simulink model "actrec_export"  (R2013a)
settings: Solver=FixedStepDiscrete  SolverMode=SingleTasking  StartTime=0  StopTime=220  RelTol=1e-3
libraries: simulink x2, dspsigops x2, dspstat3 x2, dspspect3 x2
settings Model: Creator=laurenz  LastModifiedBy=laurenz
settings OptimizationCC: OptimizeModelRefInitCode=on  LifeSpan=1
settings HardwareCC: ProdLargestAtomicInteger=Long  ProdLargestAtomicFloat=Double  ProdEndianess=LittleEndian  ProdHWDeviceType=ARM Compatible->ARM Cortex  TargetLargestAtomicInteger=Long  TargetLargestAtomicFloat=Double  TargetEndianess=LittleEndian  TargetHWDeviceType=ARM Compatible->ARM Cortex
settings RTWCC: SystemTargetFile=ert.tlc  GenCodeOnly=on  GenerateMakefile=off  TemplateMakefile=ert_default_tmf  Description=Embedded Coder  ProcessScript=ert_make_rtw_hook
settings CodeAppCC: IgnoreCustomStorageClasses=off
settings ERTTargetCC: GenerateSampleERTMain=off  IncludeMdlTerminateFcn=off  IncludeFileDelimiter=UseQuote  InlinedParameterPlacement=Hierarchical  ERTCustomFileTemplate=example_file_process.tlc  GlobalDataDefinition=InSourceFile  GlobalDataReference=InSourceFile  ERTFilePackagingFormat=Compact

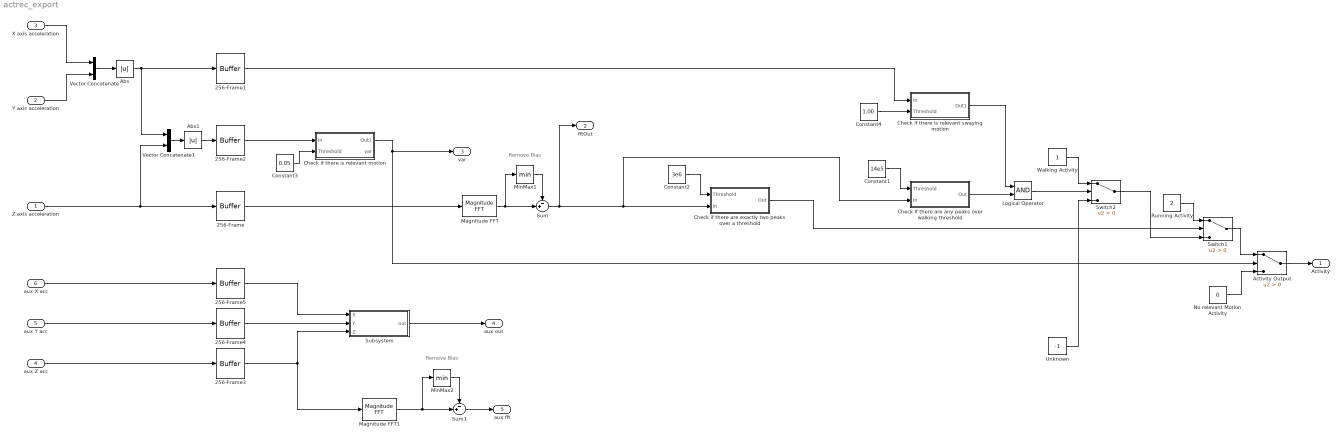
== system actrec_export ==
  note: Remove Bias
  note: Remove Bias
  Z axis acceleration : Inport  SampleTime=1
  Y axis acceleration : Inport  Port=2  SampleTime=1
  X axis acceleration : Inport  Port=3  SampleTime=1
  aux Z acc : Inport  Port=4  SampleTime=1
  aux Y acc : Inport  Port=5  SampleTime=1
  aux X acc : Inport  Port=6  SampleTime=1
  256-Frame{,1..5} (6 alike) : Buffer  N=256  V=256-64  TreatMby1Signals=One channel
  Abs : Abs
  Abs1 : Abs
  Activity Output : Switch  Criteria=u2 > Threshold
  Check if there are any peaks over walking threshold : Subsystem
  Check if there are exactly two peaks over a threshold : Subsystem
  Check if there is relevant motion : Subsystem
  Check if there is relevant swaying motion : Subsystem
  Constant1 : Constant  Value=14e5
  Constant2 : Constant  Value=3e6
  Constant3 : Constant  Value=0.05
  Constant4 : Constant  Value=1.00
  Logical Operator : Logic  AllPortsSameDT=off  OutDataTypeStr=boolean
  Magnitude FFT : dspspect3/Magnitude FFT  mag_or_magsq=Magnitude squared  FFTImplementation=Auto  fftLenInherit=on  fftsize=256
  Magnitude FFT1 : dspspect3/Magnitude FFT  mag_or_magsq=Magnitude squared  FFTImplementation=Auto  fftLenInherit=on  fftsize=256
  MinMax1 : MinMax
  MinMax2 : MinMax
  No relevant Motion Activity : Constant  Value=0
  Running Activity : Constant  Value=2
  Subsystem : Subsystem
  Sum : Sum  Inputs=-+|
  Sum1 : Sum  Inputs=-+|
  Switch1 : Switch  Criteria=u2 > Threshold
  Switch2 : Switch  Criteria=u2 > Threshold
  Unknown : Constant  Value=-1
  Vector Concatenate : Concatenate
  Vector Concatenate1 : Concatenate
  Walking Activity : Constant
  Activity : Outport
  fftOut : Outport  Port=2  PortDimensions=256
  var : Outport  Port=3
  aux out : Outport  Port=4
  aux fft : Outport  Port=5
  wires:
  Z axis acceleration/1 -> Vector Concatenate1/2, 256-Frame/1
  Activity Output/1 -> Activity/1
  No relevant Motion Activity/1 -> Activity Output/3
  Magnitude FFT/1 -> Sum/2, MinMax1/1
  MinMax1/1 -> Sum/1
  Check if there are exactly two peaks over a threshold/1(Out) -> Switch1/2
  Constant2/1 -> Check if there are exactly two peaks over a threshold/1(Threshold)
  Running Activity/1 -> Switch1/1
  Switch1/1 -> Activity Output/1
  Constant1/1 -> Check if there are any peaks over walking threshold/1(Threshold)
  Switch2/1 -> Switch1/3
  Walking Activity/1 -> Switch2/1
  Logical Operator/1 -> Switch2/2
  Check if there are any peaks over walking threshold/1(Out) -> Logical Operator/2
  Check if there is relevant swaying motion/1(Out1) -> Logical Operator/1
  Abs/1 -> 256-Frame1/1, Vector Concatenate1/1
  Vector Concatenate/1 -> Abs/1
  X axis acceleration/1 -> Vector Concatenate/1
  Y axis acceleration/1 -> Vector Concatenate/2
  Vector Concatenate1/1 -> Abs1/1
  Abs1/1 -> 256-Frame2/1
  Constant3/1 -> Check if there is relevant motion/2(Threshold)
  256-Frame2/1 -> Check if there is relevant motion/1(In)
  Constant4/1 -> Check if there is relevant swaying motion/2(Threshold)
  Check if there is relevant motion/1(Out1) -> var/1, Activity Output/2
  256-Frame/1 -> Magnitude FFT/1
  Unknown/1 -> Switch2/3
  aux Z acc/1 -> 256-Frame3/1
  aux Y acc/1 -> 256-Frame4/1
  aux X acc/1 -> 256-Frame5/1
  Subsystem/1(out) -> aux out/1
  Magnitude FFT1/1 -> MinMax2/1, Sum1/2
  MinMax2/1 -> Sum1/1
  Sum1/1 -> aux fft/1
  256-Frame5/1 -> Subsystem/1(X)
  256-Frame4/1 -> Subsystem/2(Y)
  256-Frame3/1 -> Subsystem/3(Z), Magnitude FFT1/1
  Sum/1 -> Check if there are any peaks over walking threshold/2(In), Check if there are exactly two peaks over a threshold/2(In), fftOut/1
  256-Frame1/1 -> Check if there is relevant swaying motion/1(In)

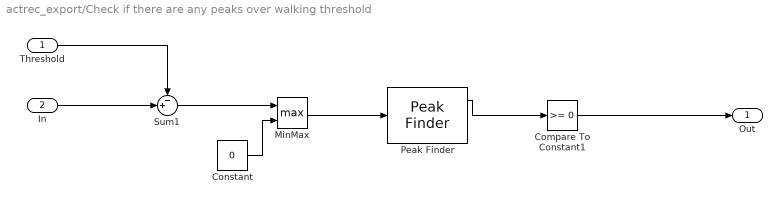
== system actrec_export/Check if there are any peaks over walking threshold ==
  Threshold : Inport
  In : Inport  Port=2
  Compare To Constant1 : simulink/Logic and Bit Operations/Compare To Constant  relop=>=  const=0  OutDataTypeStr=boolean
  Constant : Constant  Value=0
  MinMax : MinMax  Function=max  Inputs=2
  Peak Finder : dspsigops/Peak Finder  polarity=Maxima  outputIdx=off  outputVal=on  maxPeaks=10  NoiseDistinguish=off  thresh=0  roundingMode=Floor  overflowMode=off
      settings: allowOverrides=off
  Sum1 : Sum  Inputs=-+|
  Out : Outport
  wires:
  Threshold/1 -> Sum1/1
  In/1 -> Sum1/2
  Sum1/1 -> MinMax/1
  Compare To Constant1/1 -> Out/1
  Peak Finder/1 -> Compare To Constant1/1
  MinMax/1 -> Peak Finder/1
  Constant/1 -> MinMax/2

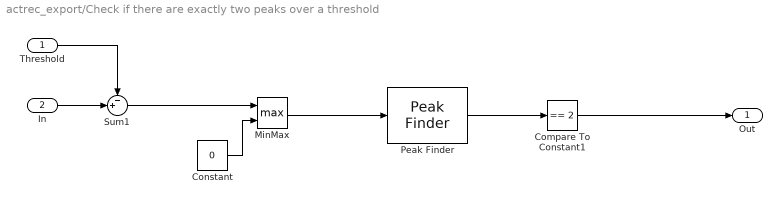
== system actrec_export/Check if there are exactly two peaks over a threshold ==
  Threshold : Inport
  In : Inport  Port=2
  Compare To Constant1 : simulink/Logic and Bit Operations/Compare To Constant  relop===  const=2  OutDataTypeStr=boolean
  Constant : Constant  Value=0
  MinMax : MinMax  Function=max  Inputs=2
  Peak Finder : dspsigops/Peak Finder  polarity=Maxima  outputIdx=off  outputVal=off  maxPeaks=10  NoiseDistinguish=on  thresh=1e6  roundingMode=Floor  overflowMode=off
      settings: allowOverrides=off
  Sum1 : Sum  Inputs=-+|
  Out : Outport
  wires:
  Threshold/1 -> Sum1/1
  In/1 -> Sum1/2
  Compare To Constant1/1 -> Out/1
  Peak Finder/1 -> Compare To Constant1/1
  Sum1/1 -> MinMax/1
  MinMax/1 -> Peak Finder/1
  Constant/1 -> MinMax/2

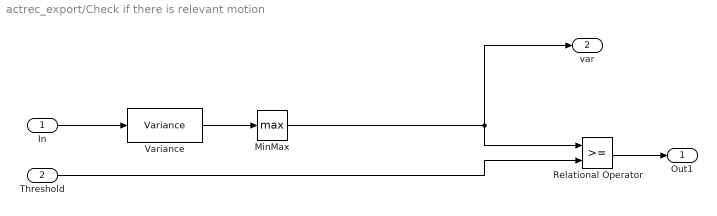
== system actrec_export/Check if there is relevant motion ==
  In : Inport
  Threshold : Inport  Port=2  PortDimensions=1
  MinMax : MinMax  Function=max
  Relational Operator : RelationalOperator
  Variance : dspstat3/Variance  run=off  reset_popup=None  InputProcessing=Columns as channels (frame based)  directionMode=Entire input  dimension=1  treatSBRowAsCol=on  roiEnable=off  roiType=Rectangles  roiPortion=Entire ROI  roiOutput=Individual statistics for each ROI  roiFlag=off  roundingMode=Floor  overflowMode=off
  Out1 : Outport  OutDataTypeStr=boolean
  var : Outport  Port=2
  wires:
  Variance/1 -> MinMax/1
  Relational Operator/1 -> Out1/1
  Threshold/1 -> Relational Operator/2
  In/1 -> Variance/1
  MinMax/1 -> Relational Operator/1, var/1

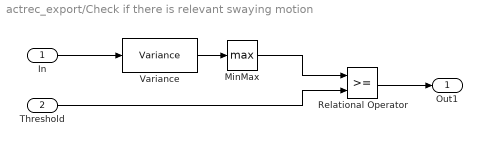
== system actrec_export/Check if there is relevant swaying motion ==
  In : Inport
  Threshold : Inport  Port=2
  MinMax : MinMax  Function=max
  Relational Operator : RelationalOperator  OutDataTypeStr=boolean
  Variance : dspstat3/Variance  run=off  reset_popup=None  InputProcessing=Columns as channels (frame based)  directionMode=Entire input  dimension=1  treatSBRowAsCol=on  roiEnable=off  roiType=Rectangles  roiPortion=Entire ROI  roiOutput=Individual statistics for each ROI  roiFlag=off  roundingMode=Floor  overflowMode=off
  Out1 : Outport
  wires:
  MinMax/1 -> Relational Operator/1
  Threshold/1 -> Relational Operator/2
  Relational Operator/1 -> Out1/1
  Variance/1 -> MinMax/1
  In/1 -> Variance/1

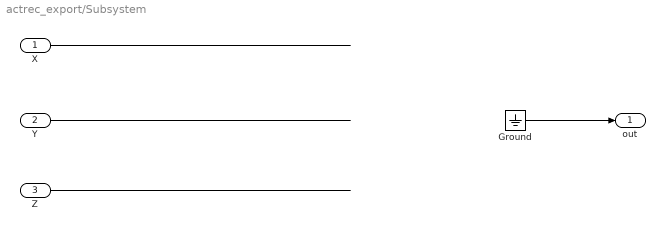
== system actrec_export/Subsystem ==
  X : Inport  SampleTime=1
  Y : Inport  Port=2  SampleTime=1
  Z : Inport  Port=3  SampleTime=1
  Ground : Ground
  out : Outport
  wires:
  X/1 -> ?
  Y/1 -> ?
  Z/1 -> ?
  Ground/1 -> out/1
